simulink model "MSFartoystyring_heading"  (Simulink 8.1)
settings: Solver=ode45  StartTime=tstart  StopTime=4000  RelTol=1e-3
values from neighbouring files (symbols this model uses):
  c = 0    [task1.m]    (also in task_1_4.m = 1)
  nc = 7.3    [task1.m]    (also in task_1_4.m)
  psi0 = 0    [task1.m]    (also in task_1_4.m)
  r0 = 0    [task1.m]    (also in task_1_4.m)
  tsamp = 1    [task1.m]    (also in task_1_4.m = 10)
  v0 = [0.001 0]'    [task1.m]    (also in task_1_4.m = [6.63 0]')
undefined symbols (not defined in the file or in its folder): msfartoystyring
undefined symbols (not defined in the file): p0
settings Model: Creator=christh  LastModifiedBy=Mat  ExtModeAutoUpdateStatusClock=off
settings OptimizationCC: InitFltsAndDblsToZero=on
settings GRTTargetCC: CodeReplacementLibrary=None  CPPClassGenCompliant=on

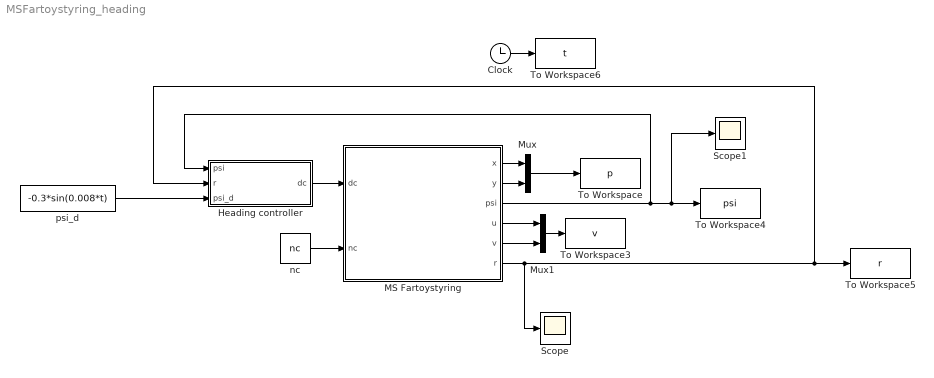
== system MSFartoystyring_heading ==
  Clock : Clock
  Heading controller : Subsystem
  MS Fartoystyring : Subsystem  mask(MS Fartoystyring for Assignment 3 G&C){x0=p0(1), y0=p0(2), u0=v0(1), v0=v0(2), psi0=psi0, r0=r0, c=c}
      mask prompts: x0 "x(t0) (m)"; y0 "y(t0) (m)"; u0 "u(t0) (m/s)"; v0 "v(t0) (m/s)"; psi0 "psi(t0) (rad)"; r0 "r(t0) (rad/s)"; c "current (0 or 1)"
      mask help:
      | Block corresponding to Figure 1 in the assignment text. Gives the response of the ship.
      |
      | The design speed of MS Fartoystyring is u=8.23 m/s.
      |
      | Input:
      | dc: commanded rudder (rad), dmax=25*pi/180
      | nc: commanded shaft speed (rad/s), nmax=85*2*pi/60
      |
      | Output:
      | x: north pos (m)
      | y: east pos (m)
      | u: surge (m/s)
      | v: sway (m/s)
      | psi: heading (rad)
      | r: yaw (rad/s)
      mask Help: Comments, bugs and help requests can be directed to the TA. Email on course website.
  Mux : Mux  Inputs=2
  Mux1 : Mux  Inputs=2
  Scope : Scope
  Scope1 : Scope
      settings: TimeRange=4000  YMin=0  YMax=0.7000000000000001
  To Workspace : ToWorkspace  VariableName=p  SampleTime=tsamp
  To Workspace3 : ToWorkspace  VariableName=v  SampleTime=tsamp
  To Workspace4 : ToWorkspace  VariableName=psi  SampleTime=tsamp
  To Workspace5 : ToWorkspace  VariableName=r  SampleTime=tsamp
  To Workspace6 : ToWorkspace  VariableName=t  SampleTime=tsamp
  nc : Constant  Value=nc
  "psi_d " : Constant  Value=-0.3*sin(0.008*t)
  wires:
  Clock/1 -> To Workspace6/1
  MS Fartoystyring/1(x) -> Mux/1
  MS Fartoystyring/2(y) -> Mux/2
  MS Fartoystyring/4(u) -> Mux1/1
  MS Fartoystyring/5(v) -> Mux1/2
  Mux/1 -> To Workspace/1
  Mux1/1 -> To Workspace3/1
  MS Fartoystyring/3(psi) -> Heading controller/1(psi), Scope1/1, To Workspace4/1
  MS Fartoystyring/6(r) -> Scope/1, Heading controller/2(r), To Workspace5/1
  nc/1 -> MS Fartoystyring/2(nc)
  "psi_d "/1 -> Heading controller/3(psi_d)
  Heading controller/1(dc) -> MS Fartoystyring/1(dc)

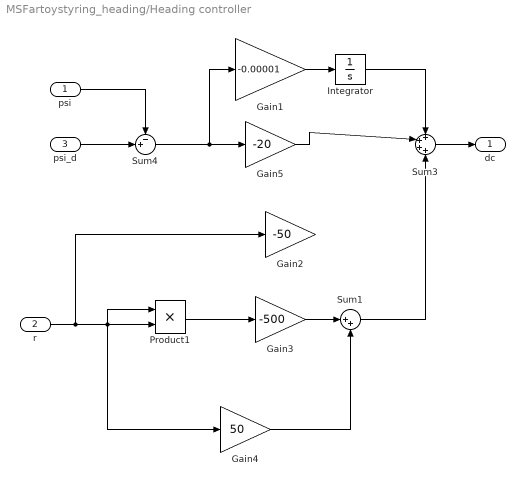
== system MSFartoystyring_heading/Heading controller ==
  psi : Inport
  r : Inport  Port=2
  psi_d : Inport  Port=3
  Gain1 : Gain  Gain=-0.00001
  Gain2 : Gain  Gain=-50
  Gain3 : Gain  Gain=-500
  Gain4 : Gain  Gain=50
  Gain5 : Gain  Gain=-20
  Integrator : Integrator
  Product1 : Product
  Sum1 : Sum  Inputs=|++
  Sum3 : Sum  Inputs=++++
  Sum4 : Sum  Inputs=-+|
  dc : Outport
  wires:
  Product1/1 -> Gain3/1
  Sum3/1 -> dc/1
  Sum4/1 -> Gain1/1, Gain5/1
  psi_d/1 -> Sum4/2
  psi/1 -> Sum4/1
  r/1 -> Gain2/1, Product1/1, Product1/2, Gain4/1
  Gain3/1 -> Sum1/1
  Gain4/1 -> Sum1/2
  Gain5/1 -> Sum3/2
  Gain1/1 -> Integrator/1
  Sum1/1 -> Sum3/4
  Integrator/1 -> Sum3/1

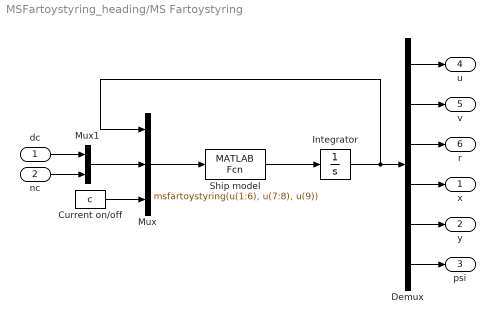
== system MSFartoystyring_heading/MS Fartoystyring ==
  dc : Inport
  nc : Inport  Port=2
  Current on/off : Constant  Value=c
  Demux : Demux  Outputs=6
  Integrator : Integrator  InitialCondition=[u0 v0 r0 x0 y0 psi0]'
  Mux : Mux  Inputs=3
  Mux1 : Mux  Inputs=2
  Ship model : MATLABFcn  MATLABFcn=msfartoystyring(u(1:6), u(7:8), u(9))  OutputDimensions=6
  x : Outport
  y : Outport  Port=2
  psi : Outport  Port=3
  u : Outport  Port=4
  v : Outport  Port=5
  r : Outport  Port=6
  wires:
  Integrator/1 -> Mux/1, Demux/1
  Mux1/1 -> Mux/2
  dc/1 -> Mux1/1
  nc/1 -> Mux1/2
  Demux/1 -> u/1
  Demux/2 -> v/1
  Demux/3 -> r/1
  Demux/4 -> x/1
  Demux/5 -> y/1
  Demux/6 -> psi/1
  Current on/off/1 -> Mux/3
  Ship model/1 -> Integrator/1
  Mux/1 -> Ship model/1
